simulink model "tri76"  (R2016b)
settings: Solver=VariableStepAuto  StartTime=0.0  StopTime=20  RelTol=1e-3
settings Model: Creator=Admin  LastModifiedBy=Admin

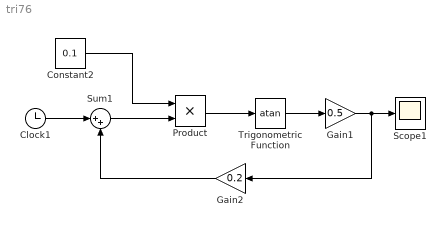
== system tri76 ==
  Clock1 : Clock
  Constant2 : Constant  Value=0.1
  Gain1 : Gain  Gain=0.5
  Gain2 : Gain  Gain=0.2
  Product : Product
  Scope1 : Scope
  Sum1 : Sum  Inputs=|++
  Trigonometric Function : Trigonometry  Operator=atan
  wires:
  Clock1/1 -> Sum1/1
  Sum1/1 -> Product/2
  Constant2/1 -> Product/1
  Gain1/1 -> Gain2/1, Scope1/1
  Gain2/1 -> Sum1/2
  Trigonometric Function/1 -> Gain1/1
  Product/1 -> Trigonometric Function/1
